simulink model "formation_planner_exp_cs_old"  (R2022b)
settings: Solver=ode5  StartTime=0.0  StopTime=80  FixedStep=1/1000  RelTol=1e-3
PreLoadFcn:
  | mbxruntime.callbacks.PreLoadFcn(bdroot);
PostLoadFcn:
  | mbxruntime.callbacks.PostLoadFcn(bdroot);
InitFcn:
  | mbxruntime.callbacks.InitFcn(bdroot);
StartFcn:
  | mbxruntime.callbacks.StartFcn(bdroot);
StopFcn:
  | mbxruntime.callbacks.StopFcn(bdroot);
model workspace (MAT data in the model file):
  mbox_table : object (value not decoded)
  model_closed = 0
  sim_status = 0
values from neighbouring files (symbols this model uses):
  c_factor = 43.75    [emplanner_init.m]
  car1_s = -10    [emplanner_init.m]
  car2_s = -20    [emplanner_init.m]
  cf = -175016    [emplanner_init.m]
  cr = -130634    [emplanner_init.m]
  KD_PID_distance = 0.0    (= 0)    [emplanner_init.m]
  KD_PID_speed = 0    [emplanner_init.m]
  KI_PID_distance = 0.0    (= 0)    [emplanner_init.m]
  KI_PID_speed = 0    [emplanner_init.m]
  KP_PID_distance = 0.5    [emplanner_init.m]
  KP_PID_speed = 1.8    [emplanner_init.m]
  la = 1.265    [emplanner_init.m]
  lb = 2.947-1.265    (= 1.682)    [emplanner_init.m]
  leader_global_kappa = global_kappa    [kappa.m]    (also in leader_global_path.mat = [0 0 0 0 0 0 0 0 0 0 0 0 ... (801 elements, 801x1)])
  leader_global_path_x = x_orgin.Data    [kappa.m]    (also in leader_global_path.mat = [2.22044604925e-16 0.999382255067 1.99750536558 2.9943522493)
  leader_global_path_y = y.Data    [kappa.m]    (also in leader_global_path.mat = [2 2 2 2 2 2 2 2 2 2 2 2 ... (801 elements, 801x1)])
  leader_global_yaw = yaw.Data    [kappa.m]    (also in leader_global_path.mat = [0 0 0 0 0 0 0 0 0 0 0 0 ... (801 elements, 801x1)])
  LQR_K1 = k(:,1)'    [emplanner_init.m]
  LQR_K2 = k(:,2)'    [emplanner_init.m]
  LQR_K3 = k(:,3)'    [emplanner_init.m]
  LQR_K4 = k(:,4)'    [emplanner_init.m]
  m = 2020    [emplanner_init.m]
  rack_displacement = [-39.14 , -37.2 , -35.29 , -33.43 , -31.6 , -29.81 , -28.06 , -26.34 , -24.66 ,      -23.01 , -21.38 , -19.79 , -18.23 , -16.69 , -15.18 , -13.7 , -12.23 , -10.8 , -9.38 , -7.98 ,     -6.61 , -5.25 , -3.91 , -2.59 , -1.29 , 0 , 1.27 , 2.54 , 3.78 , 5.02 , 6.24 , 7.46 , 8.66 ,      9.86 , 11.05 , 12.24 , 13.41 , 14.59 , 15.76 , 16.92 , 18.09 , 19.25 , 20.42 , 21.59 , 22.76 ,      23.93 , 25.11 , 26 ...(+26 chars)    [emplanner_init.m]
  right_wheel_ground = [-70 ,-67.2 , -64.4 , -61.6 , -58.8 , -56 , -53.2 , -50.4 , -47.6 , -44.8 , -42 ,      -39.2 , -36.4 , -33.6 , -30.8 , -28 , -25.2 , -22.4 , -19.6 , -16.8 , -14 , -11.2 , -8.4 , -5.6 ,      -2.8 , 0 , 2.8 , 5.6 , 8.4 , 11.2 , 14 , 16.8 , 19.6 , 22.4 , 25.2 , 28 , 30.8 , 33.6 , 36.4 ,      39.2 , 42 , 44.8 , 47.6 , 50.4 , 53.2 , 56 , 58.8 , 61.6 , 64.4 , 67.2 , 70 ]    [emplanner_init.m]
  vx_break_point = zeros(1,5000)    [emplanner_init.m]
undefined symbols (not defined in the file or in its folder): aubr, car1_global_kappa, car1_global_path_x, car1_global_path_y, car1_global_yaw, car2_global_kappa, car2_global_path_x, car2_global_path_y, car2_global_yaw, DiscIntNeverNeededParam, tablebr, vubr, warningInitialVelocity, x0
libraries: PreScanSimulinkLibrary x65, simulink x19, simulink_extras x14, Solver_SF x2
(part 20 of 31)

== matlab function formation_planner_exp_cs_old/Audi_A8_Sedan_2/PathFollower_Preview_1/LateralController/CTRL REFERENCES/Find Reference Point (pref0) on Trajectory closest to P0 Point (p0)/eml_find_closest_trajectory_points0 ==
  data: pvp input size=2; Actor_traj_distance output; TrajOffset_x_y_Y input size=3; ActorOffset_Left_Right input; p0 input size=3; Traj_x parameter; Traj_y parameter; Actor_traj_angle output; RefreshCounter parameter
function [Actor_traj_distance,Actor_traj_angle]  = eml_find_closest_trajectory_points0(pvp,TrajOffset_x_y_Y,ActorOffset_Left_Right,p0,Traj_x,Traj_y,RefreshCounter)

[Actor_traj_distance,Actor_traj_angle]  = emlfcn_find_closest_trajectory_points0(pvp,TrajOffset_x_y_Y,ActorOffset_Left_Right,p0,Traj_x,Traj_y,RefreshCounter);

% end function

== matlab function formation_planner_exp_cs_old/Global_Planner/Path planning/Path Planner Car2_0/obs/MATLAB Function2 ==
  data: x_set input; match_point_index_set output; y_set input; frenet_path_x input; frenet_path_y input; frenet_path_heading input; frenet_path_kappa input; proj_x_set output; proj_y_set output; proj_heading_set output; proj_kappa_set output
function [match_point_index_set,proj_x_set, proj_y_set,proj_heading_set,proj_kappa_set] = ...
    fcn(x_set,y_set,frenet_path_x,frenet_path_y,frenet_path_heading,frenet_path_kappa)
%该函数将批量计算x_set，y_set中的xy，在frenet_path下的投影的信息
%输入 x_set,y_set，待投影的点的集合
%x_set,y_set,frenet_path_x,frenet_path_y,frenet_path_heading,frenet_path_kappa
%曲线在直角坐标系下的x，y，heading，kappa
%输出：match_point_index_set 匹配点在frenet_path下的编号的集合(即从全局路径第一个点开始数，第几个点是匹配点)
%     proj_x y heading kappa 投影的x,y,heading,kappa的集合

% 由于事先不知道x_set中到底有多少个点需要投影，因此事先声明一个最大的数量的点作为缓冲
n = 128;
% 并且由于不知道投影点的个数，所以也不知道输出的个数，因此输出也要做缓冲，用nan表示不存在的点
% 输出最多输出128个
% 输出初始化
match_point_index_set = ones(n,1) * nan;
proj_x_set = ones(n,1) * nan;
proj_y_set = ones(n,1) * nan;
proj_heading_set = ones(n,1) * nan;
proj_kappa_set = ones(n,1) * nan;

% 找匹配点，需要利用上一个周期的结果作为下一个周期遍历的起点，因此需要声明两个全局变量

persistent is_first_run;
persistent pre_match_point_index_set;%bug :pre_match_point_index(i) 未必代表的是第i个障碍物的match_point_index
persistent pre_frenet_path_x;
persistent pre_frenet_path_y;
persistent pre_frenet_path_heading;
persistent pre_frenet_path_kappa;
persistent pre_x_set;
persistent pre_y_set;
%算法主函数入口

if isempty(is_first_run)
    %该if分支表示函数首次运行
    is_first_run = 0;
    pre_frenet_path_x = frenet_path_x;
    pre_frenet_path_y = frenet_path_y;
    pre_frenet_path_heading = frenet_path_heading;
    pre_frenet_path_kappa = frenet_path_kappa;
    %要记录首次运行计算的匹配点的结果供下个周期运行，先初始化
    pre_match_point_index_set = ones(n,1) * nan;
    %对x_set,y_set的点做遍历，找到他们的匹配点
    for i = 1 : length(x_set)
        if isnan(x_set(i))
            break;
        end
        %首次运行时，没有任何提示，只能从frenet path的第一个点开始找
        start_search_index = 1;
        % 声明increase_count，用于表示在遍历时distance连续增加的个数
        increase_count = 0;
        % 开始遍历
        min_distance = inf;
        for j = start_search_index : length(frenet_path_x)
            distance = (x_set(i) - frenet_path_x(j))^2 + (y_set(i) - frenet_path_y(j))^2;
            if distance < min_distance
                min_distance = distance;
                match_point_index_set(i) = j;
                increase_count = 0;
            else
                increase_count = increase_count + 1;
            end
            %如果distance连续增加50次就不要再遍历了，节省时间
            if increase_count > 50
                break;
            end
        end
        
        %如何通过匹配点计算投影点，请参见《自动驾驶控制算法第七讲》
        %或《自动驾驶决策规划算法》第一章第三节
        
        %取出匹配点的编号
        match_point_index = match_point_index_set(i);
        %取出匹配点的信息
        match_point_x = frenet_path_x(match_point_index);
        match_point_y = frenet_path_y(match_point_index);
        match_point_heading = frenet_path_heading(match_point_index);
        match_point_kappa = frenet_path_kappa(match_point_index);
        %计算匹配点的方向向量与法向量
        vector_match_point = [match_point_x;match_point_y];
        vector_match_point_direction = [cos(match_point_heading);sin(match_point_heading)];
        %声明待投影点的位矢
        vector_r = [x_set(i);y_set(i)];
        
       %通过匹配点计算投影点
       vector_d = vector_r - vector_match_point;
       ds = vector_d' * vector_match_point_direction;
       vector_proj_point = vector_match_point + ds * vector_match_point_direction;
       proj_heading = match_point_heading + match_point_kappa * ds;
       proj_kappa = match_point_kappa;
       %计算结果输出
       proj_x_set(i) = vector_proj_point(1);
       proj_y_set(i) = vector_proj_point(2);
       proj_heading_set(i) = proj_heading;
       proj_kappa_set(i) = proj_kappa;
    end
    %匹配点的计算结果保存，供下一个周期使用
    pre_match_point_index_set = match_point_index_set;
    pre_x_set = x_set;
    pre_y_set = y_set;
else
    %此if分支表示不是首次运行
    %对每个x_set上的点做处理
    for i = 1 : length(x_set)
        %不是首次运行，对于点x_set(i),y_set(i)来说,start_search_index =
        %pre_match_point_index_set(i)
        start_search_index = pre_match_point_index_set(i);%上个周期匹配点的编号作为本周期搜索的起点
        % 判断帧与帧之间的障碍物是否为同一个
        square_dis = (x_set(i) - pre_x_set(i))^2 + (y_set(i) - pre_y_set(i))^2;
        if square_dis > 36
            % 帧与帧之间的物体的位置距离过大，认为是两个障碍物
            start_search_index = nan;
        end
        % 声明increase_count，用于表示在遍历时distance连续增加的个数
        %%%%%%%%%
        %对于障碍物检测而言，当感知第一次检测到障碍物时，算法并不是首次运行，此时 
        %pre_match_point_index_set的值是nan，如果还用上一时刻的结果作为本周期搜索的起点
        %必然会出问题，所以要修改
        % 声明increase_count_limit
        increase_count_limit = 5;
        if isnan(start_search_index)
            %没有上个周期的结果，那就不能只检查5次了
            increase_count_limit = 50;
            %搜索起点也要设为1
            start_search_index = 1;
        end
        increase_count = 0;
        % 开始遍历
        %这里多一个步骤，判断遍历的方向
        %计算上个周期匹配点的位矢
        vector_pre_match_point = [pre_frenet_path_x(start_search_index);pre_frenet_path_y(start_search_index)];
        vector_pre_match_point_direction = ...
            [cos(pre_frenet_path_heading(start_search_index));sin(pre_frenet_path_heading(start_search_index))];
        %判断遍历的方向
        flag = ([x_set(i);y_set(i)] - vector_pre_match_point)' * vector_pre_match_point_direction;
        min_distance = inf;
        if flag > 0.001
            for j = start_search_index : length(frenet_path_x)
                distance = (x_set(i) - frenet_path_x(j))^2 + (y_set(i) - frenet_path_y(j))^2;
                if distance < min_distance
                    min_distance = distance;
                    match_point_index_set(i) = j;
                    increase_count = 0;
                else
                    increase_count = increase_count + 1;
                end
                %如果distance连续增加increase_count_limit次就不要再遍历了，节省时间
                if increase_count > increase_count_limit
                    break;
                end
            end
        elseif flag < - 0.001
            for j = start_search_index : -1 : 1
                distance = (x_set(i) - frenet_path_x(j))^2 + (y_set(i) - frenet_path_y(j))^2;
                if distance < min_distance
                    min_distance = distance;
                    match_point_index_set(i) = j;
                    increase_count = 0;
                else
                    increase_count = increase_count + 1;
                end
                %如果distance连续增加increase_count_limit次就不要再遍历了，节省时间
                if increase_count > increase_count_limit
                    break;
                end
            end
        else
            match_point_index_set(i) = start_search_index;
        end
        
        %如何通过匹配点计算投影点，请参见《自动驾驶控制算法第七讲》
        %或《自动驾驶决策规划算法》第一章第三节
        
        %取出匹配点的编号
        match_point_index = match_point_index_set(i);
        %取出匹配点的信息
        match_point_x = frenet_path_x(match_point_index);
        match_point_y = frenet_path_y(match_point_index);
        match_point_heading = frenet_path_heading(match_point_index);
        match_point_kappa = frenet_path_kappa(match_point_index);
        %计算匹配点的方向向量与法向量
        vector_match_point = [match_point_x;match_point_y];
        vector_match_point_direction = [cos(match_point_heading);sin(match_point_heading)];
        %声明待投影点的位矢
        vector_r = [x_set(i);y_set(i)];
        
       %通过匹配点计算投影点
       vector_d = vector_r - vector_match_point;
       ds = vector_d' * vector_match_point_direction;
       vector_proj_point = vector_match_point + ds * vector_match_point_direction;
       proj_heading = match_point_heading + match_point_kappa * ds;
       proj_kappa = match_point_kappa;
       %计算结果输出
       proj_x_set(i) = vector_proj_point(1);
       proj_y_set(i) = vector_proj_point(2);
       proj_heading_set(i) = proj_heading;
       proj_kappa_set(i) = proj_kappa;
  
    end
    %匹配点的计算结果保存，供下一个周期使用
    pre_match_point_index_set = match_point_index_set;
    pre_frenet_path_x = frenet_path_x;
    pre_frenet_path_y = frenet_path_y;
    pre_frenet_path_heading = frenet_path_heading;
    pre_frenet_path_kappa = frenet_path_kappa;
    pre_x_set = x_set;
    pre_y_set = y_set;
end

== matlab function formation_planner_exp_cs_old/Global_Planner/perception module/MATLAB Function1 ==
  data: obs_x_set_init input; obs_x_set output; obs_y_set_init input; obs_vel_set_init input; obs_heading_set_init input; car1_x input; car1_y input; car2_x input; car2_y input; obs_y_set output; obs_vel_set output; obs_heading_set output
function [obs_x_set,obs_y_set,obs_vel_set,obs_heading_set] = fcn(obs_x_set_init,obs_y_set_init,obs_vel_set_init,obs_heading_set_init,car1_x,car1_y,car2_x,car2_y)


obs_x_set = ones(32,1)*nan;
obs_y_set = ones(32,1)*nan;
obs_vel_set = ones(32,1)*nan;
obs_heading_set = ones(32,1)*nan;
count = 1;
for i = 1:length(obs_x_set_init)
    if(isnan(obs_x_set_init))
        break;
    else
        len_car1 = (obs_x_set_init(i)-car1_x)^2+(obs_y_set_init(i)-car1_y)^2;
        len_car2 = (obs_x_set_init(i)-car2_x)^2+(obs_y_set_init(i)-car2_y)^2;
        if((len_car1>3) && (len_car2>3))
            obs_x_set(count) = obs_x_set_init(i);
            obs_y_set(count) = obs_y_set_init(i);
            obs_vel_set(count) = obs_vel_set_init(i);
            obs_heading_set(count) = obs_heading_set_init(i);
            count = count +1;
        end
    end
end

== matlab function formation_planner_exp_cs_old/Global_Planner/Path planning/EM Planner/obs/MATLAB Function ==
  data: obs_x_set_gcs input; static_obs_x_set output; obs_y_set_gcs input; obs_heading_set_gcs input; obs_velocity_set_gcs input; static_obs_y_set output; dynamic_obs_x_set output; dynamic_obs_y_set output; dynamic_obs_vx_set output; dynamic_obs_vy_set output
function [static_obs_x_set,static_obs_y_set,dynamic_obs_x_set,dynamic_obs_y_set,dynamic_obs_vx_set,dynamic_obs_vy_set]...
    = fcn(obs_x_set_gcs,obs_y_set_gcs,obs_heading_set_gcs,obs_velocity_set_gcs)

%该函数将分类静态障碍物和动态障碍物
%输出初始化
n = 32;
static_obs_x_set = ones(n,1)*nan;
static_obs_y_set = ones(n,1)*nan;
dynamic_obs_x_set = ones(n,1)*nan;
dynamic_obs_y_set = ones(n,1)*nan;
dynamic_obs_vx_set = ones(n,1)*nan;
dynamic_obs_vy_set = ones(n,1)*nan;
count_static = 1;
count_dynamic = 1;
for i = 1:length(obs_x_set_gcs)
    if isnan(obs_velocity_set_gcs(i))
        break;
    end
    if abs(obs_velocity_set_gcs(i)) < 0.1
        static_obs_x_set(count_static) = obs_x_set_gcs(i);
        static_obs_y_set(count_static) = obs_y_set_gcs(i);
        count_static = count_static + 1;
    else
        dynamic_obs_x_set(count_dynamic) = obs_x_set_gcs(i);
        dynamic_obs_y_set(count_dynamic) = obs_y_set_gcs(i);
        dynamic_obs_vx_set(count_dynamic) = obs_velocity_set_gcs(i)*cos(obs_heading_set_gcs(i));
        dynamic_obs_vy_set(count_dynamic) = obs_velocity_set_gcs(i)*sin(obs_heading_set_gcs(i));
        count_dynamic = count_dynamic + 1;      
    end
end

== matlab function formation_planner_exp_cs_old/Global_Planner/Path planning/EM Planner/obs/MATLAB Function1 ==
  data: x_set input; match_point_index_set output; y_set input; frenet_path_x input; frenet_path_y input; frenet_path_heading input; frenet_path_kappa input; proj_x_set output; proj_y_set output; proj_heading_set output; proj_kappa_set output
function [match_point_index_set,proj_x_set, proj_y_set,proj_heading_set,proj_kappa_set] = ...
    fcn(x_set,y_set,frenet_path_x,frenet_path_y,frenet_path_heading,frenet_path_kappa)
%该函数将批量计算x_set，y_set中的xy，在frenet_path下的投影的信息
%输入 x_set,y_set，待投影的点的集合
%x_set,y_set,frenet_path_x,frenet_path_y,frenet_path_heading,frenet_path_kappa
%曲线在直角坐标系下的x，y，heading，kappa
%输出：match_point_index_set 匹配点在frenet_path下的编号的集合(即从全局路径第一个点开始数，第几个点是匹配点)
%     proj_x y heading kappa 投影的x,y,heading,kappa的集合

% 由于事先不知道x_set中到底有多少个点需要投影，因此事先声明一个最大的数量的点作为缓冲
n = 128;
% 并且由于不知道投影点的个数，所以也不知道输出的个数，因此输出也要做缓冲，用nan表示不存在的点
% 输出最多输出128个
% 输出初始化
match_point_index_set = ones(n,1) * nan;
proj_x_set = ones(n,1) * nan;
proj_y_set = ones(n,1) * nan;
proj_heading_set = ones(n,1) * nan;
proj_kappa_set = ones(n,1) * nan;

% 找匹配点，需要利用上一个周期的结果作为下一个周期遍历的起点，因此需要声明两个全局变量

persistent is_first_run;
persistent pre_match_point_index_set;%bug :pre_match_point_index(i) 未必代表的是第i个障碍物的match_point_index
persistent pre_frenet_path_x;
persistent pre_frenet_path_y;
persistent pre_frenet_path_heading;
persistent pre_frenet_path_kappa;
persistent pre_x_set;
persistent pre_y_set;
%算法主函数入口

if isempty(is_first_run)
    %该if分支表示函数首次运行
    is_first_run = 0;
    pre_frenet_path_x = frenet_path_x;
    pre_frenet_path_y = frenet_path_y;
    pre_frenet_path_heading = frenet_path_heading;
    pre_frenet_path_kappa = frenet_path_kappa;
    %要记录首次运行计算的匹配点的结果供下个周期运行，先初始化
    pre_match_point_index_set = ones(n,1) * nan;
    %对x_set,y_set的点做遍历，找到他们的匹配点
    for i = 1 : length(x_set)
        if isnan(x_set(i))
            break;
        end
        %首次运行时，没有任何提示，只能从frenet path的第一个点开始找
        start_search_index = 1;
        % 声明increase_count，用于表示在遍历时distance连续增加的个数
        increase_count = 0;
        % 开始遍历
        min_distance = inf;
        for j = start_search_index : length(frenet_path_x)
            distance = (x_set(i) - frenet_path_x(j))^2 + (y_set(i) - frenet_path_y(j))^2;
            if distance < min_distance
                min_distance = distance;
                match_point_index_set(i) = j;
                increase_count = 0;
            else
                increase_count = increase_count + 1;
            end
            %如果distance连续增加50次就不要再遍历了，节省时间
            if increase_count > 50
                break;
            end
        end
        
        %如何通过匹配点计算投影点，请参见《自动驾驶控制算法第七讲》
        %或《自动驾驶决策规划算法》第一章第三节
        
        %取出匹配点的编号
        match_point_index = match_point_index_set(i);
        %取出匹配点的信息
        match_point_x = frenet_path_x(match_point_index);
        match_point_y = frenet_path_y(match_point_index);
        match_point_heading = frenet_path_heading(match_point_index);
        match_point_kappa = frenet_path_kappa(match_point_index);
        %计算匹配点的方向向量与法向量
        vector_match_point = [match_point_x;match_point_y];
        vector_match_point_direction = [cos(match_point_heading);sin(match_point_heading)];
        %声明待投影点的位矢
        vector_r = [x_set(i);y_set(i)];
        
       %通过匹配点计算投影点
       vector_d = vector_r - vector_match_point;
       ds = vector_d' * vector_match_point_direction;
       vector_proj_point = vector_match_point + ds * vector_match_point_direction;
       proj_heading = match_point_heading + match_point_kappa * ds;
       proj_kappa = match_point_kappa;
       %计算结果输出
       proj_x_set(i) = vector_proj_point(1);
       proj_y_set(i) = vector_proj_point(2);
       proj_heading_set(i) = proj_heading;
       proj_kappa_set(i) = proj_kappa;
    end
    %匹配点的计算结果保存，供下一个周期使用
    pre_match_point_index_set = match_point_index_set;
    pre_x_set = x_set;
    pre_y_set = y_set;
else
    %此if分支表示不是首次运行
    %对每个x_set上的点做处理
    for i = 1 : length(x_set)
        %不是首次运行，对于点x_set(i),y_set(i)来说,start_search_index =
        %pre_match_point_index_set(i)
        start_search_index = pre_match_point_index_set(i);%上个周期匹配点的编号作为本周期搜索的起点
        % 判断帧与帧之间的障碍物是否为同一个
        square_dis = (x_set(i) - pre_x_set(i))^2 + (y_set(i) - pre_y_set(i))^2;
        if square_dis > 36
            % 帧与帧之间的物体的位置距离过大，认为是两个障碍物
            start_search_index = nan;
        end
        % 声明increase_count，用于表示在遍历时distance连续增加的个数
        %%%%%%%%%
        %对于障碍物检测而言，当感知第一次检测到障碍物时，算法并不是首次运行，此时 
        %pre_match_point_index_set的值是nan，如果还用上一时刻的结果作为本周期搜索的起点
        %必然会出问题，所以要修改
        % 声明increase_count_limit
        increase_count_limit = 5;
        if isnan(start_search_index)
            %没有上个周期的结果，那就不能只检查5次了
            increase_count_limit = 50;
            %搜索起点也要设为1
            start_search_index = 1;
        end
        increase_count = 0;
        % 开始遍历
        %这里多一个步骤，判断遍历的方向
        %计算上个周期匹配点的位矢
        vector_pre_match_point = [pre_frenet_path_x(start_search_index);pre_frenet_path_y(start_search_index)];
        vector_pre_match_point_direction = ...
            [cos(pre_frenet_path_heading(start_search_index));sin(pre_frenet_path_heading(start_search_index))];
        %判断遍历的方向
        flag = ([x_set(i);y_set(i)] - vector_pre_match_point)' * vector_pre_match_point_direction;
        min_distance = inf;
        if flag > 0.001
            for j = start_search_index : length(frenet_path_x)
                distance = (x_set(i) - frenet_path_x(j))^2 + (y_set(i) - frenet_path_y(j))^2;
                if distance < min_distance
                    min_distance = distance;
                    match_point_index_set(i) = j;
                    increase_count = 0;
                else
                    increase_count = increase_count + 1;
                end
                %如果distance连续增加increase_count_limit次就不要再遍历了，节省时间
                if increase_count > increase_count_limit
                    break;
                end
            end
        elseif flag < - 0.001
            for j = start_search_index : -1 : 1
                distance = (x_set(i) - frenet_path_x(j))^2 + (y_set(i) - frenet_path_y(j))^2;
                if distance < min_distance
                    min_distance = distance;
                    match_point_index_set(i) = j;
                    increase_count = 0;
                else
                    increase_count = increase_count + 1;
                end
                %如果distance连续增加increase_count_limit次就不要再遍历了，节省时间
                if increase_count > increase_count_limit
                    break;
                end
            end
        else
            match_point_index_set(i) = start_search_index;
        end
        
        %如何通过匹配点计算投影点，请参见《自动驾驶控制算法第七讲》
        %或《自动驾驶决策规划算法》第一章第三节
        
        %取出匹配点的编号
        match_point_index = match_point_index_set(i);
        %取出匹配点的信息
        match_point_x = frenet_path_x(match_point_index);
        match_point_y = frenet_path_y(match_point_index);
        match_point_heading = frenet_path_heading(match_point_index);
        match_point_kappa = frenet_path_kappa(match_point_index);
        %计算匹配点的方向向量与法向量
        vector_match_point = [match_point_x;match_point_y];
        vector_match_point_direction = [cos(match_point_heading);sin(match_point_heading)];
        %声明待投影点的位矢
        vector_r = [x_set(i);y_set(i)];
        
       %通过匹配点计算投影点
       vector_d = vector_r - vector_match_point;
       ds = vector_d' * vector_match_point_direction;
       vector_proj_point = vector_match_point + ds * vector_match_point_direction;
       proj_heading = match_point_heading + match_point_kappa * ds;
       proj_kappa = match_point_kappa;
       %计算结果输出
       proj_x_set(i) = vector_proj_point(1);
       proj_y_set(i) = vector_proj_point(2);
       proj_heading_set(i) = proj_heading;
       proj_kappa_set(i) = proj_kappa;
  
    end
    %匹配点的计算结果保存，供下一个周期使用
    pre_match_point_index_set = match_point_index_set;
    pre_frenet_path_x = frenet_path_x;
    pre_frenet_path_y = frenet_path_y;
    pre_frenet_path_heading = frenet_path_heading;
    pre_frenet_path_kappa = frenet_path_kappa;
    pre_x_set = x_set;
    pre_y_set = y_set;
end

== matlab function formation_planner_exp_cs_old/Global_Planner/Path planning/EM Planner/obs/MATLAB Function2 ==
  data: x_set input; match_point_index_set output; y_set input; frenet_path_x input; frenet_path_y input; frenet_path_heading input; frenet_path_kappa input; proj_x_set output; proj_y_set output; proj_heading_set output; proj_kappa_set output
function [match_point_index_set,proj_x_set, proj_y_set,proj_heading_set,proj_kappa_set] = ...
    fcn(x_set,y_set,frenet_path_x,frenet_path_y,frenet_path_heading,frenet_path_kappa)
%该函数将批量计算x_set，y_set中的xy，在frenet_path下的投影的信息
%输入 x_set,y_set，待投影的点的集合
%x_set,y_set,frenet_path_x,frenet_path_y,frenet_path_heading,frenet_path_kappa
%曲线在直角坐标系下的x，y，heading，kappa
%输出：match_point_index_set 匹配点在frenet_path下的编号的集合(即从全局路径第一个点开始数，第几个点是匹配点)
%     proj_x y heading kappa 投影的x,y,heading,kappa的集合

% 由于事先不知道x_set中到底有多少个点需要投影，因此事先声明一个最大的数量的点作为缓冲
n = 128;
% 并且由于不知道投影点的个数，所以也不知道输出的个数，因此输出也要做缓冲，用nan表示不存在的点
% 输出最多输出128个
% 输出初始化
match_point_index_set = ones(n,1) * nan;
proj_x_set = ones(n,1) * nan;
proj_y_set = ones(n,1) * nan;
proj_heading_set = ones(n,1) * nan;
proj_kappa_set = ones(n,1) * nan;

% 找匹配点，需要利用上一个周期的结果作为下一个周期遍历的起点，因此需要声明两个全局变量

persistent is_first_run;
persistent pre_match_point_index_set;%bug :pre_match_point_index(i) 未必代表的是第i个障碍物的match_point_index
persistent pre_frenet_path_x;
persistent pre_frenet_path_y;
persistent pre_frenet_path_heading;
persistent pre_frenet_path_kappa;
persistent pre_x_set;
persistent pre_y_set;
%算法主函数入口

if isempty(is_first_run)
    %该if分支表示函数首次运行
    is_first_run = 0;
    pre_frenet_path_x = frenet_path_x;
    pre_frenet_path_y = frenet_path_y;
    pre_frenet_path_heading = frenet_path_heading;
    pre_frenet_path_kappa = frenet_path_kappa;
    %要记录首次运行计算的匹配点的结果供下个周期运行，先初始化
    pre_match_point_index_set = ones(n,1) * nan;
    %对x_set,y_set的点做遍历，找到他们的匹配点
    for i = 1 : length(x_set)
        if isnan(x_set(i))
            break;
        end
        %首次运行时，没有任何提示，只能从frenet path的第一个点开始找
        start_search_index = 1;
        % 声明increase_count，用于表示在遍历时distance连续增加的个数
        increase_count = 0;
        % 开始遍历
        min_distance = inf;
        for j = start_search_index : length(frenet_path_x)
            distance = (x_set(i) - frenet_path_x(j))^2 + (y_set(i) - frenet_path_y(j))^2;
            if distance < min_distance
                min_distance = distance;
                match_point_index_set(i) = j;
                increase_count = 0;
            else
                increase_count = increase_count + 1;
            end
            %如果distance连续增加50次就不要再遍历了，节省时间
            if increase_count > 50
                break;
            end
        end
        
        %如何通过匹配点计算投影点，请参见《自动驾驶控制算法第七讲》
        %或《自动驾驶决策规划算法》第一章第三节
        
        %取出匹配点的编号
        match_point_index = match_point_index_set(i);
        %取出匹配点的信息
        match_point_x = frenet_path_x(match_point_index);
        match_point_y = frenet_path_y(match_point_index);
        match_point_heading = frenet_path_heading(match_point_index);
        match_point_kappa = frenet_path_kappa(match_point_index);
        %计算匹配点的方向向量与法向量
        vector_match_point = [match_point_x;match_point_y];
        vector_match_point_direction = [cos(match_point_heading);sin(match_point_heading)];
        %声明待投影点的位矢
        vector_r = [x_set(i);y_set(i)];
        
       %通过匹配点计算投影点
       vector_d = vector_r - vector_match_point;
       ds = vector_d' * vector_match_point_direction;
       vector_proj_point = vector_match_point + ds * vector_match_point_direction;
       proj_heading = match_point_heading + match_point_kappa * ds;
       proj_kappa = match_point_kappa;
       %计算结果输出
       proj_x_set(i) = vector_proj_point(1);
       proj_y_set(i) = vector_proj_point(2);
       proj_heading_set(i) = proj_heading;
       proj_kappa_set(i) = proj_kappa;
    end
    %匹配点的计算结果保存，供下一个周期使用
    pre_match_point_index_set = match_point_index_set;
    pre_x_set = x_set;
    pre_y_set = y_set;
else
    %此if分支表示不是首次运行
    %对每个x_set上的点做处理
    for i = 1 : length(x_set)
        %不是首次运行，对于点x_set(i),y_set(i)来说,start_search_index =
        %pre_match_point_index_set(i)
        start_search_index = pre_match_point_index_set(i);%上个周期匹配点的编号作为本周期搜索的起点
        % 判断帧与帧之间的障碍物是否为同一个
        square_dis = (x_set(i) - pre_x_set(i))^2 + (y_set(i) - pre_y_set(i))^2;
        if square_dis > 36
            % 帧与帧之间的物体的位置距离过大，认为是两个障碍物
            start_search_index = nan;
        end
        % 声明increase_count，用于表示在遍历时distance连续增加的个数
        %%%%%%%%%
        %对于障碍物检测而言，当感知第一次检测到障碍物时，算法并不是首次运行，此时 
        %pre_match_point_index_set的值是nan，如果还用上一时刻的结果作为本周期搜索的起点
        %必然会出问题，所以要修改
        % 声明increase_count_limit
        increase_count_limit = 5;
        if isnan(start_search_index)
            %没有上个周期的结果，那就不能只检查5次了
            increase_count_limit = 50;
            %搜索起点也要设为1
            start_search_index = 1;
        end
        increase_count = 0;
        % 开始遍历
        %这里多一个步骤，判断遍历的方向
        %计算上个周期匹配点的位矢
        vector_pre_match_point = [pre_frenet_path_x(start_search_index);pre_frenet_path_y(start_search_index)];
        vector_pre_match_point_direction = ...
            [cos(pre_frenet_path_heading(start_search_index));sin(pre_frenet_path_heading(start_search_index))];
        %判断遍历的方向
        flag = ([x_set(i);y_set(i)] - vector_pre_match_point)' * vector_pre_match_point_direction;
        min_distance = inf;
        if flag > 0.001
            for j = start_search_index : length(frenet_path_x)
                distance = (x_set(i) - frenet_path_x(j))^2 + (y_set(i) - frenet_path_y(j))^2;
                if distance < min_distance
                    min_distance = distance;
                    match_point_index_set(i) = j;
                    increase_count = 0;
                else
                    increase_count = increase_count + 1;
                end
                %如果distance连续增加increase_count_limit次就不要再遍历了，节省时间
                if increase_count > increase_count_limit
                    break;
                end
            end
        elseif flag < - 0.001
            for j = start_search_index : -1 : 1
                distance = (x_set(i) - frenet_path_x(j))^2 + (y_set(i) - frenet_path_y(j))^2;
                if distance < min_distance
                    min_distance = distance;
                    match_point_index_set(i) = j;
                    increase_count = 0;
                else
                    increase_count = increase_count + 1;
                end
                %如果distance连续增加increase_count_limit次就不要再遍历了，节省时间
                if increase_count > increase_count_limit
                    break;
                end
            end
        else
            match_point_index_set(i) = start_search_index;
        end
        
        %如何通过匹配点计算投影点，请参见《自动驾驶控制算法第七讲》
        %或《自动驾驶决策规划算法》第一章第三节
        
        %取出匹配点的编号
        match_point_index = match_point_index_set(i);
        %取出匹配点的信息
        match_point_x = frenet_path_x(match_point_index);
        match_point_y = frenet_path_y(match_point_index);
        match_point_heading = frenet_path_heading(match_point_index);
        match_point_kappa = frenet_path_kappa(match_point_index);
        %计算匹配点的方向向量与法向量
        vector_match_point = [match_point_x;match_point_y];
        vector_match_point_direction = [cos(match_point_heading);sin(match_point_heading)];
        %声明待投影点的位矢
        vector_r = [x_set(i);y_set(i)];
        
       %通过匹配点计算投影点
       vector_d = vector_r - vector_match_point;
       ds = vector_d' * vector_match_point_direction;
       vector_proj_point = vector_match_point + ds * vector_match_point_direction;
       proj_heading = match_point_heading + match_point_kappa * ds;
       proj_kappa = match_point_kappa;
       %计算结果输出
       proj_x_set(i) = vector_proj_point(1);
       proj_y_set(i) = vector_proj_point(2);
       proj_heading_set(i) = proj_heading;
       proj_kappa_set(i) = proj_kappa;
  
    end
    %匹配点的计算结果保存，供下一个周期使用
    pre_match_point_index_set = match_point_index_set;
    pre_frenet_path_x = frenet_path_x;
    pre_frenet_path_y = frenet_path_y;
    pre_frenet_path_heading = frenet_path_heading;
    pre_frenet_path_kappa = frenet_path_kappa;
    pre_x_set = x_set;
    pre_y_set = y_set;
end

== matlab function formation_planner_exp_cs_old/Global_Planner/Path planning/EM Planner/obs/obs filter ==
  data: host_x input; obs_x_set_final output; host_y input; host_heading_xy input; obs_x_set_gcs input; obs_y_set_gcs input; obs_velocity_set_gcs input; obs_heading_set_gcs input; obs_y_set_final output; obs_velocity_set_final output; obs_heading_set_final output
function [obs_x_set_final,obs_y_set_final,obs_velocity_set_final,obs_heading_set_final] = fcn(host_x,host_y,host_heading_xy,obs_x_set_gcs,obs_y_set_gcs,obs_velocity_set_gcs,obs_heading_set_gcs)
% 该函数将筛选障碍物，纵向[-10,60] 横向[-10,10]的障碍物才会被考虑
% 该函数只是一种单车道的临时办法，考虑到多车道情况，即使障碍物距离较远也应该考虑
% EM Planner完全体是多车道并行计算的，每个车道都生成参考线然后并行计算出多条轨迹，再选择最优的轨迹作为输出

%传感器最多可以识别32个障碍物
n = 32;
%输出初始化
obs_x_set_final = ones(n,1)*nan;
obs_y_set_final = ones(n,1)*nan;
obs_velocity_set_final = ones(n,1)*nan;
obs_heading_set_final = ones(n,1)*nan;
count = 1;
for i = 1:length(obs_x_set_gcs)
    if isnan(obs_x_set_gcs(i))
        break;
    end
    %自车的heading的方向向量与法向量
    tor = [cos(host_heading_xy);sin(host_heading_xy)];
    nor = [-sin(host_heading_xy);cos(host_heading_xy)];
    %障碍物与自车的距离向量
    vector_obs = [obs_x_set_gcs(i);obs_y_set_gcs(i)] - [host_x;host_y];
    %障碍物纵向距离
    lon_distance = vector_obs'*tor;
    %障碍物横向距离
    lat_distance = vector_obs'*nor;
    
    if (lon_distance < 60) && (lon_distance > -10) && (lat_distance > -25) && (lat_distance < 25)
        obs_x_set_final(count) = obs_x_set_gcs(i);
        obs_y_set_final(count) = obs_y_set_gcs(i);
        obs_heading_set_final(count) = obs_heading_set_gcs(i);
        obs_velocity_set_final(count) = obs_velocity_set_gcs(i);
        count = count + 1;
    end
end

== matlab function formation_planner_exp_cs_old/Global_Planner/Path planning/EM Planner/obs/visual obs filter ==
  data: host_speed input; static_obs_s_set_init input; static_obs_s_set output; static_obs_l_set_init input; dynamic_obs_s_set_init input; dynamic_obs_l_set_init input; dynamic_obs_s_dot_set_init input; dynamic_obs_l_dot_set_init input; static_obs_l_set output; dynamic_obs_x_set output; dynamic_obs_y_set output; dynamic_obs_vx_set output; dynamic_obs_vy_set output; dynamic_obs_x_set_init input; dynamic_obs_y_set_init input; dynamic_obs_vx_set_init input; dynamic_obs_vy_set_init input
function [static_obs_s_set,static_obs_l_set,dynamic_obs_x_set,dynamic_obs_y_set,dynamic_obs_vx_set,dynamic_obs_vy_set] = ...
    fcn(host_speed,static_obs_s_set_init,static_obs_l_set_init,dynamic_obs_s_set_init,dynamic_obs_l_set_init,dynamic_obs_s_dot_set_init,dynamic_obs_l_dot_set_init,dynamic_obs_x_set_init,dynamic_obs_y_set_init,dynamic_obs_vx_set_init,dynamic_obs_vy_set_init)

n = 0;
for i = 1 :length(dynamic_obs_s_set_init)
    if(isnan(dynamic_obs_s_set_init(i)))
        break;
    else
        n=n+1;
    end
end
m = 0;
for i = 1 :length(static_obs_s_set_init)
    if(isnan(static_obs_s_set_init(i)))
        break;
    else
        m=m+1;
    end
end

visual_flag = zeros(n,1);
visual_count = 0;
for i = 1:n
    if isnan(dynamic_obs_s_set_init(i))
        break;
    end
    if abs(dynamic_obs_l_dot_set_init(i)) < 0.3
        % 侧向缓慢移动的障碍物
        if abs(dynamic_obs_l_set_init(i)) > 2
            continue;
        else
            if(dynamic_obs_s_dot_set_init(i)>=host_speed)
                continue;
            else
                visual_flag(i) = 1;
                visual_count = visual_count+1;
            end
        end
    end
end

static_obs_s_set = ones(128,1) * nan;
static_obs_l_set = ones(128,1) * nan;
dynamic_obs_x_set = ones(128,1) * nan;
dynamic_obs_y_set = ones(128,1) * nan;
dynamic_obs_vx_set = ones(128,1) * nan;
dynamic_obs_vy_set = ones(128,1) * nan;
static_obs_s_set = static_obs_s_set_init;
static_obs_l_set = static_obs_l_set_init;

static_count = m+1;
dynamic_count = 1;
for i = 1:n
    if(visual_flag(i)==1)
        t = dynamic_obs_s_set_init(i)/(host_speed-dynamic_obs_s_dot_set_init(i));
        static_obs_s_set(static_count) = dynamic_obs_s_set_init(i)+t*dynamic_obs_s_dot_set_init(i);
        static_obs_l_set(static_count) = dynamic_obs_l_set_init(i)+t*dynamic_obs_l_dot_set_init(i);
        static_count = static_count+1;
    else
        dynamic_obs_x_set(dynamic_count) = dynamic_obs_x_set_init(i);
        dynamic_obs_y_set(dynamic_count) = dynamic_obs_y_set_init(i); 
        dynamic_obs_vx_set(dynamic_count) = dynamic_obs_vx_set_init(i);
        dynamic_obs_vy_set(dynamic_count) = dynamic_obs_vy_set_init(i);
        dynamic_count = dynamic_count +1 ;
    end
end

== matlab function formation_planner_exp_cs_old/Global_Planner/Path planning/EM Planner/generate convex space ==
  data: dp_speed_s input; s_lb output; dp_speed_t input; path_index2s input; obs_st_s_in_set input; obs_st_s_out_set input; obs_st_t_in_set input; obs_st_t_out_set input; s_ub output; s_dot_lb output; s_dot_ub output; trajectory_kappa_init input; max_lateral_accel input
function [s_lb,s_ub,s_dot_lb,s_dot_ub] = fcn(dp_speed_s,dp_speed_t,path_index2s,obs_st_s_in_set,obs_st_s_out_set,...
    obs_st_t_in_set,obs_st_t_out_set,trajectory_kappa_init,max_lateral_accel)
% 该函数将计算出s,s_dot的上下界，开辟凸空间供二次规划使用
% dp_speed_s t 最多有16个，输出初始化n = 16
n = 16;
s_lb = ones(n,1)*-inf;
s_ub = ones(n,1)*inf;
s_dot_lb = ones(n,1)*-inf;
s_dot_ub = ones(n,1)*inf;
path_index2s_end_index = length(path_index2s);
dp_speed_end_index = length(dp_speed_s);

% path_index2s也是有缓冲的，找到有效的path_index2s的末尾的位置，赋值给path_index2s_end_index
for k = 2:length(path_index2s)
    if path_index2s(k) == 0 && path_index2s(k-1) ~= 0
        path_index2s_end_index = k - 1;
        break;
    end
    path_index2s_end_index = k;
end
% 找到dp_speed_s中有效的位置，赋值给dp_speed_end_index
for k = 1:length(dp_speed_s)
    if isnan(dp_speed_s(k))
        dp_speed_end_index = k - 1;
        break;
    end
end

for i = 1:n
    % 该循环将施加车辆动力学约束
    if isnan(dp_speed_s(i))
        break;
    end
    cur_s = dp_speed_s(i);
    % 通过插值的方式找到cur_s 所对应的曲率
    cur_kappa = interp1(path_index2s(1:path_index2s_end_index),trajectory_kappa_init(1:path_index2s_end_index),cur_s);
    % a = v^2 * k => v^2 = a/k 注意除0保护
    max_speed =  sqrt(max_lateral_accel / (abs(cur_kappa) + 1e-10));
    min_speed = 0;
    s_dot_lb(i) = min_speed;
    s_dot_ub(i) = max_speed;    
end



for i = 1:length(obs_st_s_in_set)
    if isnan(obs_st_s_in_set(i))
        continue;
    end
    % 取s t 直线的中点，作为obs_s obs_t 的坐标 
    obs_t = (obs_st_t_in_set(i) + obs_st_t_out_set(i)) / 2;
    obs_s = (obs_st_s_in_set(i) + obs_st_s_out_set(i)) / 2;
    % 计算障碍物的纵向速度
    obs_speed = (obs_st_s_out_set(i) - obs_st_s_in_set(i)) / (obs_st_t_out_set(i) - obs_st_t_in_set(i));
    % 插值找到当t = obs_t时，dp_speed_s 的值
    dp_s = interp1([0;dp_speed_t(1:dp_speed_end_index)],[0;dp_speed_s(1:dp_speed_end_index)],obs_t);
    % 找到dp_speed_t中 与obs_st_t_in_set(i)最近的时间，并将此时间的编号赋值给t_lb_index
    for j = 1:length(dp_speed_t) - 1
        if dp_speed_t(1) > obs_st_t_in_set(i)
            % 如果障碍物切入时间比0.5秒还要短，那么t_lb_index = 1
            break;
        elseif dp_speed_t(j) <= obs_st_t_in_set(i) && dp_speed_t(j + 1) > obs_st_t_in_set(i)
            % 否则遍历dp_speed_t 找到与obs_st_t_in_set(i)最近的点的编号
            break;
        end
    end
    t_lb_index = j;% 将点的编号赋值给j
     % 找到dp_speed_t中 与obs_st_t_out_set(i)最近的时间，并将此时间的编号赋值给t_ub_index
    for j = 1:length(dp_speed_t) - 1
        if dp_speed_t(1) > obs_st_t_out_set(i)
            break;
        elseif dp_speed_t(j) <= obs_st_t_out_set(i) && dp_speed_t(j + 1) > obs_st_t_out_set(i)
            break;
        end
    end
    t_ub_index = j;
    % 这里稍微做个缓冲，把 t_lb_index 稍微缩小一些，t_ub_index稍微放大一些
    t_lb_index = max(t_lb_index - 2,3);% 最低为3 因为碰瓷没法处理
    t_ub_index = min(t_ub_index + 2,dp_speed_end_index);
    if obs_s > dp_s
        % 决策为减速避让
        for m = t_lb_index:t_ub_index
            % 在t_lb_index:t_ub_index的区间上 s的上界不可以超过障碍物st斜直线
            dp_t = dp_speed_t(m);
            s_ub(m) = min(s_ub(m),obs_st_s_in_set(i) + obs_speed * (dp_t - obs_st_t_in_set(i)));
        end
    else 
        % 决策为加速超车
        for m = t_lb_index:t_ub_index
             % 在t_lb_index:t_ub_index的区间上 s的下界不能小于障碍物st斜直线
            dp_t = dp_speed_t(m);
            s_lb(m) = max(s_lb(m),obs_st_s_in_set(i) + obs_speed * (dp_t - obs_st_t_in_set(i)));
        end
    end
        
end

== matlab function formation_planner_exp_cs_old/Audi_A8_Sedan_3/control module1/control main/chassic steering system/MATLAB Function ==
  data: u input; right_steer output; la input; lb input
function right_steer = fcn(u,la,lb)
if abs(u)<1e-2
   right_steer = u;
else
   R =  (la+lb)/tan(u);
   right_steer = atan((la+lb)/(R+1.624/2));
end

== matlab function formation_planner_exp_cs_old/Global_Planner/Path planning/EM Planner/generate st graph ==
  data: pre_trajectory_s input; obs_st_s_in_set output; pre_trajectory_t input; dynamic_obs_s_set input; dynamic_obs_l_set input; dynamic_obs_s_dot_set input; dynamic_obs_l_dot_set input; obs_st_s_out_set output; obs_st_t_in_set output; obs_st_t_out_set output
function [obs_st_s_in_set,obs_st_s_out_set,obs_st_t_in_set,obs_st_t_out_set] = ...
    fcn(pre_trajectory_s,pre_trajectory_t,dynamic_obs_s_set,dynamic_obs_l_set,dynamic_obs_s_dot_set,dynamic_obs_l_dot_set)
% 该函数将生成st图，使用斜直线模型
n = length(dynamic_obs_s_set);
% 输出初始化
obs_st_s_in_set = ones(n,1) * nan;
obs_st_s_out_set = ones(n,1) * nan;
obs_st_t_in_set = ones(n,1) * nan;
obs_st_t_out_set = ones(n,1) * nan;
obs_st_l_in_set = ones(n,1) * nan;
obs_st_l_out_set = ones(n,1) * nan;

for i = 1:length(dynamic_obs_s_set)
    if isnan(dynamic_obs_s_set(i))
        break;
    end
    if abs(dynamic_obs_l_dot_set(i)) < 0.3
        % 侧向缓慢移动的障碍物
        if abs(dynamic_obs_l_set(i)) > 2
            % 距离横向太远，速度规划直接忽略
            continue;
        else
            % TODO需要做虚拟障碍物
            % 这里由于算力原因没做逻辑
            % 如何做：感知模块加逻辑，给出障碍物跟踪，判断两帧之间的感知所看到的障碍物是否为同一个
            %         速度规划模块在一开始先给出虚拟障碍物决策，不做处理
            %         下一帧，路径规划拿到虚拟障碍物标记，规划出绕过去的路径/跟车路径
            %                 速度规划计算出速度，绕过去/跟车
            % 本算法欠缺的：障碍物结构体 结构体不仅要包含坐标 速度 还要包含 决策标记(是否为虚拟障碍物，左绕还是右绕，避让还是超车)
            %              感知模块，判断两帧之间的障碍物是否为同一个
            %              算力
            continue;
        end
    end
    % t_zero 为动态障碍物的l到0，所需要的时间
    t_zero = - dynamic_obs_l_set(i) / dynamic_obs_l_dot_set(i); % 时间等于路程除以速度
    % 计算+-2缓冲时间
    t_boundary1 = 2 / dynamic_obs_l_dot_set(i) + t_zero;
    t_boundary2 = -2 / dynamic_obs_l_dot_set(i) + t_zero;
    if t_boundary1 > t_boundary2
        t_max = t_boundary1;
        t_min = t_boundary2;
    else
        t_max = t_boundary2;
        t_min = t_boundary1;
    end
    if t_max < 1 || t_min > 8
        % 对于切入切出太远的，或者碰瓷的，忽略
        % 车辆运动是要受到车辆动力学制约的，如果有碰瓷的，即使规划出了很大的加速度，车辆也执行不了
        % 碰瓷障碍物也需要做虚拟障碍物和路径规划一起解决
        continue
    end
    if t_min < 0 && t_max > 0
        % 在感知看到的时候，障碍物已经在+-2的内部了
        obs_st_s_in_set(i) = dynamic_obs_s_set(i);
        % 匀速运动
        obs_st_s_out_set(i) = dynamic_obs_s_set(i) + dynamic_obs_s_dot_set(i) * t_max;
        obs_st_t_in_set(i) = 0;
        obs_st_t_out_set(i) = t_max;
    else
        % 正常障碍物
        obs_st_s_in_set(i) = dynamic_obs_s_set(i) + + dynamic_obs_s_dot_set(i) * t_min;
        obs_st_s_out_set(i) = dynamic_obs_s_set(i) + dynamic_obs_s_dot_set(i) * t_max;
        obs_st_t_in_set(i) = t_min;
        obs_st_t_out_set(i) = t_max;
    end 
end

== matlab function formation_planner_exp_cs_old/Global_Planner/Path planning/Path Planner Car2_0/obs/obs filter ==
  data: host_x input; obs_x_set_final output; host_y input; host_heading_xy input; obs_x_set_gcs input; obs_y_set_gcs input; obs_velocity_set_gcs input; obs_heading_set_gcs input; obs_y_set_final output; obs_velocity_set_final output; obs_heading_set_final output
function [obs_x_set_final,obs_y_set_final,obs_velocity_set_final,obs_heading_set_final] = fcn(host_x,host_y,host_heading_xy,obs_x_set_gcs,obs_y_set_gcs,obs_velocity_set_gcs,obs_heading_set_gcs)
% 该函数将筛选障碍物，纵向[-10,60] 横向[-10,10]的障碍物才会被考虑
% 该函数只是一种单车道的临时办法，考虑到多车道情况，即使障碍物距离较远也应该考虑
% EM Planner完全体是多车道并行计算的，每个车道都生成参考线然后并行计算出多条轨迹，再选择最优的轨迹作为输出

%传感器最多可以识别32个障碍物
n = 32;
%输出初始化
obs_x_set_final = ones(n,1)*nan;
obs_y_set_final = ones(n,1)*nan;
obs_velocity_set_final = ones(n,1)*nan;
obs_heading_set_final = ones(n,1)*nan;
count = 1;
for i = 1:length(obs_x_set_gcs)
    if isnan(obs_x_set_gcs(i))
        break;
    end
    %自车的heading的方向向量与法向量
    tor = [cos(host_heading_xy);sin(host_heading_xy)];
    nor = [-sin(host_heading_xy);cos(host_heading_xy)];
    %障碍物与自车的距离向量
    vector_obs = [obs_x_set_gcs(i);obs_y_set_gcs(i)] - [host_x;host_y];
    %障碍物纵向距离
    lon_distance = vector_obs'*tor;
    %障碍物横向距离
    lat_distance = vector_obs'*nor;
    
    if (lon_distance < 60) && (lon_distance > -10) && (lat_distance > -25) && (lat_distance < 25)
        obs_x_set_final(count) = obs_x_set_gcs(i);
        obs_y_set_final(count) = obs_y_set_gcs(i);
        obs_heading_set_final(count) = obs_heading_set_gcs(i);
        obs_velocity_set_final(count) = obs_velocity_set_gcs(i);
        count = count + 1;
    end
end

== matlab function formation_planner_exp_cs_old/Global_Planner/Path planning/Path Planner Car2_0/obs/visual obs filter ==
  data: host_speed input; static_obs_s_set_init input; static_obs_s_set output; static_obs_l_set_init input; dynamic_obs_s_set_init input; dynamic_obs_l_set_init input; dynamic_obs_s_dot_set_init input; dynamic_obs_l_dot_set_init input; static_obs_l_set output; dynamic_obs_x_set output; dynamic_obs_y_set output; dynamic_obs_vx_set output; dynamic_obs_vy_set output; dynamic_obs_x_set_init input; dynamic_obs_y_set_init input; dynamic_obs_vx_set_init input; dynamic_obs_vy_set_init input
function [static_obs_s_set,static_obs_l_set,dynamic_obs_x_set,dynamic_obs_y_set,dynamic_obs_vx_set,dynamic_obs_vy_set] = ...
    fcn(host_speed,static_obs_s_set_init,static_obs_l_set_init,dynamic_obs_s_set_init,dynamic_obs_l_set_init,dynamic_obs_s_dot_set_init,dynamic_obs_l_dot_set_init,dynamic_obs_x_set_init,dynamic_obs_y_set_init,dynamic_obs_vx_set_init,dynamic_obs_vy_set_init)

n = 0;
for i = 1 :length(dynamic_obs_s_set_init)
    if(isnan(dynamic_obs_s_set_init(i)))
        break;
    else
        n=n+1;
    end
end
m = 0;
for i = 1 :length(static_obs_s_set_init)
    if(isnan(static_obs_s_set_init(i)))
        break;
    else
        m=m+1;
    end
end

visual_flag = zeros(n,1);
visual_count = 0;
for i = 1:n
    if isnan(dynamic_obs_s_set_init(i))
        break;
    end
    if abs(dynamic_obs_l_dot_set_init(i)) < 0.3
        % 侧向缓慢移动的障碍物
        if abs(dynamic_obs_l_set_init(i)) > 2
            continue;
        else
            if(dynamic_obs_s_dot_set_init(i)>=host_speed)
                continue;
            else
                visual_flag(i) = 1;
                visual_count = visual_count+1;
            end
        end
    end
end

static_obs_s_set = ones(128,1) * nan;
static_obs_l_set = ones(128,1) * nan;
dynamic_obs_x_set = ones(128,1) * nan;
dynamic_obs_y_set = ones(128,1) * nan;
dynamic_obs_vx_set = ones(128,1) * nan;
dynamic_obs_vy_set = ones(128,1) * nan;
static_obs_s_set = static_obs_s_set_init;
static_obs_l_set = static_obs_l_set_init;

static_count = m+1;
dynamic_count = 1;
for i = 1:n
    if(visual_flag(i)==1)
        t = dynamic_obs_s_set_init(i)/(host_speed-dynamic_obs_s_dot_set_init(i));
        static_obs_s_set(static_count) = dynamic_obs_s_set_init(i)+t*dynamic_obs_s_dot_set_init(i);
        static_obs_l_set(static_count) = dynamic_obs_l_set_init(i)+t*dynamic_obs_l_dot_set_init(i);
        static_count = static_count+1;
    else
        dynamic_obs_x_set(dynamic_count) = dynamic_obs_x_set_init(i);
        dynamic_obs_y_set(dynamic_count) = dynamic_obs_y_set_init(i); 
        dynamic_obs_vx_set(dynamic_count) = dynamic_obs_vx_set_init(i);
        dynamic_obs_vy_set(dynamic_count) = dynamic_obs_vy_set_init(i);
        dynamic_count = dynamic_count +1 ;
    end
end

== matlab function formation_planner_exp_cs_old/Global_Planner/Path planning/Path Planner Car2_0/path and speed merge ==
  data: s input; trajectory_x output; s_dot input; s_dot2 input; relative_time input; current_time input; path_s input; trajectory_x_init input; trajectory_y_init input; trajectory_heading_init input; trajectory_kappa_init input; trajectory_y output; trajectory_heading output; trajectory_kappa output; trajectory_speed output; trajectory_accel output; trajectory_time output
function [trajectory_x,trajectory_y,trajectory_heading,trajectory_kappa,trajectory_speed,trajectory_accel,trajectory_time] = ...
    fcn(s,s_dot,s_dot2,relative_time,current_time,path_s,trajectory_x_init,trajectory_y_init,trajectory_heading_init,trajectory_kappa_init)
% 该函数将合并path和speed
% 由于path 是 60个点，speed 有 401个点，合并后，path和speed有401个点，因此需要做插值
n = 401;
trajectory_x = zeros(n,1);
trajectory_y = zeros(n,1);
trajectory_heading = zeros(n,1);
trajectory_kappa = zeros(n,1);
trajectory_speed = zeros(n,1);

trajectory_accel = zeros(n,1);
index = 1;
% 由于trajectory_x_init中不是所有的值都有效，(有nan) 所以要找到有效值的范围
while ~isnan(trajectory_x_init(index)) 
    index = index + 1;
end
index = index - 1;
trajectory_time = zeros(n,1);
for i = 1:n-1
    %interp1 线性插值
    % 若 x = [1,2] y = [3,4]
    %interp1(x,y,1.5) 会得到3.5
    %interp1 的缺点是 在端点或超过端点的，结果为nan
    % interp1(x,y,2) 不会等于4 而是会等于nan
    % interp1(x,y,6) 也会等于nan，所以在端点处要单独处理
    trajectory_x(i) = interp1(path_s(1:index),trajectory_x_init(1:index),s(i));
    trajectory_y(i) = interp1(path_s(1:index),trajectory_y_init(1:index),s(i));
    trajectory_heading(i) = interp1(path_s(1:index),trajectory_heading_init(1:index),s(i));
    trajectory_kappa(i) = interp1(path_s(1:index),trajectory_kappa_init(1:index),s(i));
    trajectory_time(i) = relative_time(i) + current_time;%速度规划会得到相对时间，转换成绝对时间
    trajectory_speed(i) = s_dot(i);
    trajectory_accel(i) = s_dot2(i);
end
% 端点单独处理
trajectory_x(end) = trajectory_x_init(end);
trajectory_y(end) = trajectory_y_init(end);
trajectory_heading(end) = trajectory_heading_init(end);
trajectory_kappa(end) = trajectory_kappa_init(end);
trajectory_time(end) = relative_time(end) + current_time;
trajectory_speed(end) = s_dot(end);
trajectory_accel(end) = s_dot2(end);
